simulink model "FlightController_1"  (R2022a)
settings: Solver=FixedStepAuto  StartTime=0.0  StopTime=inf  RelTol=1e-3
model workspace (MATLAB code in the model file):
  | m = 1.2;                  % mass (kg)
  | g = 9.81;                 % gravity (m/s^2)
  | I = diag([0.014,0.018,0.028]); % inertia matrix (kg·m^2)
  | l = 0.225;                % arm length (m)
  | b = 2.98e-6*(2*pi)^2;     % thrust coeff
  | d = 1.14e-7*(2*pi)^2;     % torque coeff
  | Cd = 0.1;                 % drag coeff
  | m_e = [20; 0; -40];       % earth mag field (uT)
  | wind = [0.5; 0; 0];       % constant wind (m/s)
libraries: slpidlib x6, simulink x3
settings Model: Creator=pvsha  LastModifiedBy=parv6
settings OptimizationCC: DefaultParameterBehavior=Inlined  EnhancedBackFolding=on  PassReuseOutputArgsThreshold=0  OptimizeBlockOrder=speed  DifferentSizesBufferReuse=on  OptimizationCustomize=off
settings DebuggingCC: UnderspecifiedInitializationDetection=Classic  ParameterTunabilityLossMsg=error  SFUnexpectedBacktrackingDiag=warning  SFNoUnconditionalDefaultTransitionDiag=warning
settings HardwareCC: TargetBitPerPointer=64  TargetBitPerSizeT=64  TargetBitPerPtrDiffT=64  TargetLongLongMode=on  TargetIntDivRoundTo=Zero  TargetEndianess=LittleEndian  TargetWordSize=64  TargetHWDeviceType=MATLAB Host  ProdEqTarget=off
settings ModelReferenceCC: PropagateSignalLabelsOutOfModel=off
settings SFSimCC: MATLABDynamicMemAlloc=off
settings RTWCC: Description=Generic Real-Time Target  GenCodeOnly=on  GenerateReport=on  BuildConfiguration=Debug  LaunchReport=on
settings CodeAppCC: ForceParamTrailComments=on  OperatorAnnotations=on  EnableCustomComments=on

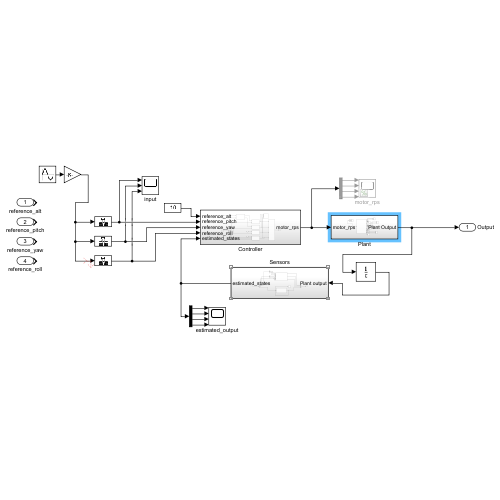
[thumbnail: Simulink's stored preview of the top-level diagram]
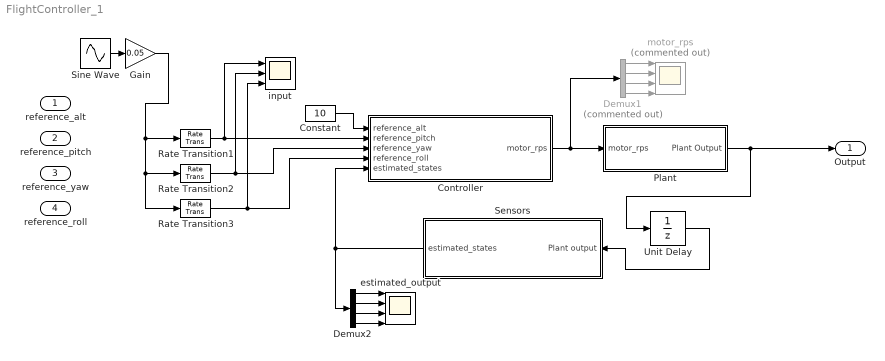
== system FlightController_1 ==
  reference_alt : Inport
  reference_pitch : Inport  Port=2
  reference_yaw : Inport  Port=3
  reference_roll : Inport  Port=4
  Constant : Constant  Value=10
  Controller : Subsystem
  Demux1 : Demux  Commented=on
  Demux2 : Demux
  Gain : Gain  Gain=0.05
  Plant : Subsystem
  Rate Transition1 : RateTransition  OutPortSampleTime=0.1
  Rate Transition2 : RateTransition  OutPortSampleTime=0.1
  Rate Transition3 : RateTransition  OutPortSampleTime=0.1
  Sensors : Subsystem
  Sine Wave : Sin  SampleTime=0
  Unit Delay : UnitDelay  SampleTime=-1  HasFrameUpgradeWarning=on
  estimated_output : Scope  NumInputPorts=4
  input : Scope  NumInputPorts=3
  motor_rps : Scope  Commented=on  NumInputPorts=4
  Output : Outport  SignalName=Output
  wires:
  Sensors/1(estimated_states) -> Demux2/1, Controller/5(estimated_states)
  Plant/1(Plant Output) -> Unit Delay/1, Output/1
  Rate Transition1/1 -> input/1, Controller/2(reference_pitch)
  Rate Transition2/1 -> input/2, Controller/3(reference_yaw)
  Rate Transition3/1 -> input/3, Controller/4(reference_roll)
  Unit Delay/1 -> Sensors/1(Plant output)
  Gain/1 -> Rate Transition3/1, Rate Transition2/1, Rate Transition1/1
  Demux1/1 -> motor_rps/1
  Demux1/3 -> motor_rps/3
  Demux1/4 -> motor_rps/4
  Demux1/2 -> motor_rps/2
  Controller/1(motor_rps) -> Demux1/1, Plant/1(motor_rps)
  Demux2/1 -> estimated_output/1
  Demux2/3 -> estimated_output/3
  Demux2/4 -> estimated_output/4
  Demux2/2 -> estimated_output/2
  Sine Wave/1 -> Gain/1
  ? -> ?
  Constant/1 -> Controller/1(reference_alt)

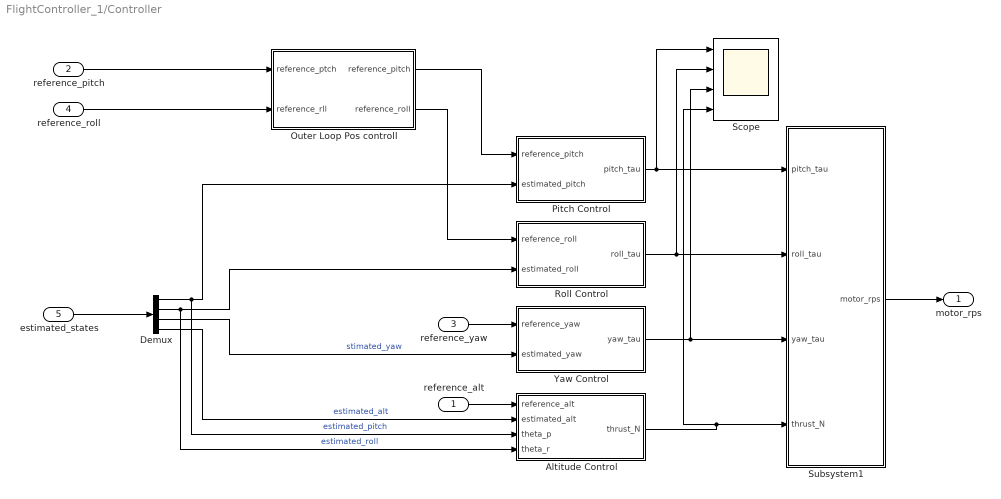
== system FlightController_1/Controller ==
  reference_alt : Inport
  reference_pitch : Inport  Port=2
  reference_yaw : Inport  Port=3
  reference_roll : Inport  Port=4
  estimated_states : Inport  Port=5  PortDimensions=4
  Altitude Control : Subsystem
  Demux : Demux
  Outer Loop Pos controll : Subsystem
  Pitch Control : Subsystem
  Roll Control : Subsystem
  Scope : Scope  NumInputPorts=4
  Subsystem1 : Subsystem
  Yaw Control : Subsystem
  motor_rps : Outport
  wires:
  estimated_states/1 -> Demux/1
  Subsystem1/1(motor_rps) -> motor_rps/1
  Pitch Control/1(pitch_tau) -> Scope/1, Subsystem1/1(pitch_tau)
  Roll Control/1(roll_tau) -> Scope/2, Subsystem1/2(roll_tau)
  Altitude Control/1(thrust_N) -> Scope/4, Subsystem1/4(thrust_N)
  reference_yaw/1 -> Yaw Control/1(reference_yaw)
  reference_pitch/1 -> Outer Loop Pos controll/1(reference_ptch)
  reference_alt/1 -> Altitude Control/1(reference_alt)
  Demux/4 -> Altitude Control/2(estimated_alt)  "estimated_alt"
  Demux/1 -> Altitude Control/3(theta_p), Pitch Control/2(estimated_pitch)  "estimated_pitch"
  Demux/2 -> Altitude Control/4(theta_r), Roll Control/2(estimated_roll)  "estimated_roll"
  Demux/3 -> Yaw Control/2(estimated_yaw)  "stimated_yaw"
  Outer Loop Pos controll/1(reference_pitch) -> Pitch Control/1(reference_pitch)
  Outer Loop Pos controll/2(reference_roll) -> Roll Control/1(reference_roll)
  reference_roll/1 -> Outer Loop Pos controll/2(reference_rll)
  Yaw Control/1(yaw_tau) -> Scope/3, Subsystem1/3(yaw_tau)

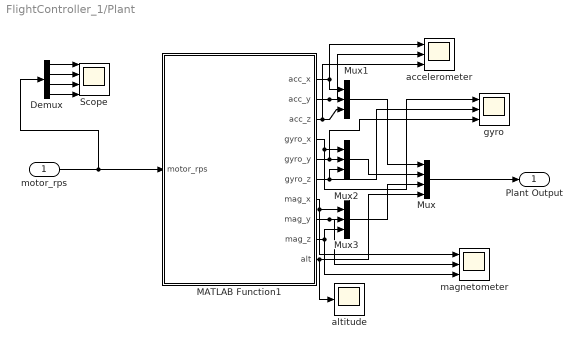
== system FlightController_1/Plant ==
  motor_rps : Inport
  Demux : Demux
  MATLAB Function1 : MATLAB Function  TreatAsAtomicUnit=on
  Mux : Mux
  Mux1 : Mux  Inputs=3
  Mux2 : Mux  Inputs=3
  Mux3 : Mux  Inputs=3
  Scope : Scope  NumInputPorts=4
  accelerometer : Scope  NumInputPorts=3
  altitude : Scope
  gyro : Scope  NumInputPorts=3
  magnetometer : Scope  NumInputPorts=3
  Plant Output : Outport
  wires:
  Mux/1 -> Plant Output/1
  motor_rps/1 -> MATLAB Function1/1(motor_rps), Demux/1
  Demux/1 -> Scope/1
  Demux/2 -> Scope/2
  Demux/3 -> Scope/3
  Demux/4 -> Scope/4
  MATLAB Function1/2(acc_y) -> accelerometer/2, Mux1/2
  MATLAB Function1/1(acc_x) -> accelerometer/1, Mux1/1
  MATLAB Function1/3(acc_z) -> Mux1/3, accelerometer/3
  MATLAB Function1/8(mag_y) -> magnetometer/2, Mux3/2
  MATLAB Function1/7(mag_x) -> magnetometer/1, Mux3/1
  MATLAB Function1/9(mag_z) -> magnetometer/3, Mux3/3
  Mux1/1 -> Mux/1
  Mux2/1 -> Mux/2
  Mux3/1 -> Mux/3
  MATLAB Function1/10(alt) -> Mux/4, altitude/1
  MATLAB Function1/6(gyro_z) -> gyro/2, Mux2/3
  MATLAB Function1/4(gyro_x) -> gyro/1, Mux2/1
  MATLAB Function1/5(gyro_y) -> gyro/3, Mux2/2

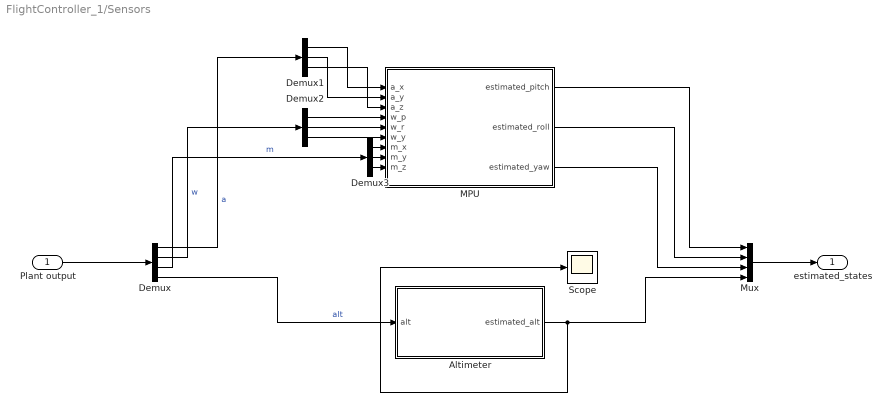
== system FlightController_1/Sensors ==
  Plant output : Inport
  Altimeter : Subsystem
  Demux : Demux
  Demux1 : Demux  Outputs=3
  Demux2 : Demux  Outputs=3
  Demux3 : Demux  Outputs=3
  MPU : Subsystem
  Mux : Mux
  Scope : Scope
  estimated_states : Outport
  wires:
  Plant output/1 -> Demux/1
  MPU/2(estimated_roll) -> Mux/2
  MPU/3(estimated_yaw) -> Mux/3
  MPU/1(estimated_pitch) -> Mux/1
  Mux/1 -> estimated_states/1
  Altimeter/1(estimated_alt) -> Scope/1, Mux/4
  Demux/1 -> Demux1/1  "a"
  Demux1/1 -> MPU/1(a_x)
  Demux1/2 -> MPU/2(a_y)
  Demux1/3 -> MPU/3(a_z)
  Demux2/2 -> MPU/5(w_r)
  Demux2/1 -> MPU/4(w_p)
  Demux2/3 -> MPU/6(w_y)
  Demux/2 -> Demux2/1  "w"
  Demux3/1 -> MPU/7(m_x)
  Demux3/2 -> MPU/8(m_y)
  Demux3/3 -> MPU/9(m_z)
  Demux/3 -> Demux3/1  "m"
  Demux/4 -> Altimeter/1(alt)  "alt"

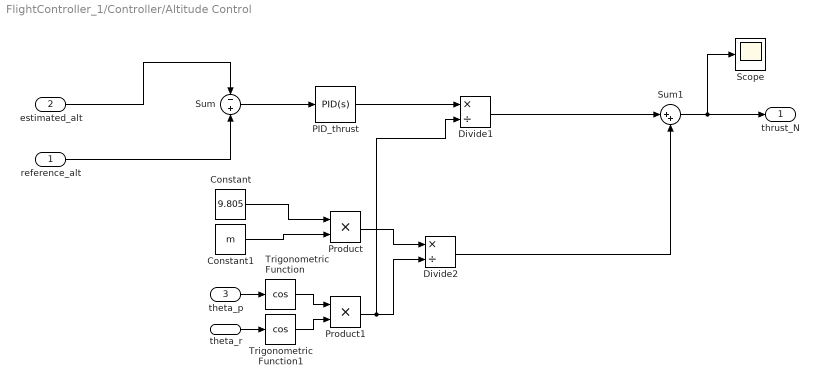
== system FlightController_1/Controller/Altitude Control ==
  reference_alt : Inport
  estimated_alt : Inport  Port=2
  theta_p : Inport  Port=3
  theta_r : Inport  Port=4
  Constant : Constant  Value=9.805
  Constant1 : Constant  Value=m
  Divide1 : Product  Inputs=*/
  Divide2 : Product  Inputs=*/
  PID_thrust : slpidlib/PID Controller  Controller=PID  Form=Parallel  TimeDomain=Continuous-time  UseExternalTs=off  SampleTime=-1  IntegratorMethod=Forward Euler  FilterMethod=Forward Euler  ControllerParametersSource=internal  P=0.8  I=0.5  UseKiTs=off  D=0  N=100  UseFilter=on  TunerSelectOption=Transfer Function Based (PID Tuner App)  InitialConditionSource=internal  InitialConditionForIntegrator=0  InitialConditionForFilter=0  DifferentiatorICPrevScaledInput=0  ExternalReset=none  TrackingMode=off  Kt=1  LimitOutput=off  SatLimitsSource=internal  UpperSaturationLimit=inf  LowerSaturationLimit=-inf  LinearizeAsGain=on  AntiWindupMode=none  Kb=1  POutMin=[]  POutMax=[]  IOutMin=[]  IOutMax=[]  DOutMin=[]  DOutMax=[]  NOutMin=[]  NOutMax=[]  SumOutMin=[]  SumOutMax=[]  SaturationOutMin=[]  SaturationOutMax=[]  PParamMin=[]  PParamMax=[]  IParamMin=[]  IParamMax=[]  DParamMin=[]  DParamMax=[]  NParamMin=[]  NParamMax=[]  KbParamMin=[]  KbParamMax=[]  KtParamMin=[]  KtParamMax=[]  KbOutMin=[]  KbOutMax=[]  KtOutMin=[]  KtOutMax=[]  IntegratorOutMin=[]  IntegratorOutMax=[]  FilterOutMin=[]  FilterOutMax=[]  SumI1OutMin=[]  SumI1OutMax=[]  SumI2OutMin=[]  SumI2OutMax=[]  SumI3OutMin=[]  SumI3OutMax=[]  SumI4OutMin=[]  SumI4OutMax=[]  SumDOutMin=[]  SumDOutMax=[]  DifferentiatorOutMin=[]  DifferentiatorOutMax=[]  FilterDiffOutCoefMin=[]  FilterDiffOutCoefMax=[]  ReciprocalOutMin=[]  ReciprocalOutMax=[]  SumDenOutMin=[]  SumDenOutMax=[]  SumNumOutMin=[]  SumNumOutMax=[]  DivideOutMin=[]  DivideOutMax=[]  UdiffTsProdOutMin=[]  UdiffTsProdOutMax=[]  NTsProdOutMin=[]  NTsProdOutMax=[]  UintegralTsProdOutMin=[]  UintegralTsProdOutMax=[]  UngainTsProdOutMin=[]  UngainTsProdOutMax=[]  ClampingZeroOutDataTypeStr=Inherit: Inherit via back propagation  ClampingZeroOutMin=[]  ClampingZeroOutMax=[]  FilterDenConstantOutDataTypeStr=Inherit: Inherit via back propagation  FilterDenConstantOutMin=[]  FilterDenConstantOutMax=[]  PCopyOutDataTypeStr=Inherit: Inherit via back propagation  PCopyOutMin=[]  PCopyOutMax=[]  NCopyOutDataTypeStr=Inherit: Inherit via back propagation  NCopyOutMin=[]  NCopyOutMax=[]  IntegratorContinuousStateAttributes=''  IntegratorStateMustResolveToSignalObject=off  IntegratorRTWStateStorageClass=Auto  FilterContinuousStateAttributes=''  FilterStateMustResolveToSignalObject=off  FilterRTWStateStorageClass=Auto  ParallelPVariant=InternalParameters  IdealPVariant=Disabled  IVariant=InternalParameters  DVariant=InternalParameters  IntegratorVariant=Continuous  SatVariant=Disabled  AWVariant=Passthrough  PCopyVariant=Disabled  TRVariant=Disabled  FdbkBlocksVariant=Forward  IdealPFdbkVariant=Disabled  SatFdbkVariant=Disabled  DerivativeFilterVariant=ContFilter  NVariant=InternalParameters  NCopyVariant=Disabled  FilterICVariant=InternalICsFilter  IntegratorICVariant=InternalICs  ExternalResetVariant=Disabled  TRSumVariant=Passthrough  SumFdbkVariant=Disabled  SumVariant=Sum_PID  TsampFilterVariant=InternalTs  TsampNgainVariant=Passthrough  TsampIntegralVariant=Passthrough  ExternalSaturationOutDataTypeStr=Inherit: Same as second input  aMode=0
  Product : Product
  Product1 : Product
  Scope : Scope
  Sum : Sum  Inputs=-+
  Sum1 : Sum  Inputs=|++
  Trigonometric Function : Trigonometry  Operator=cos
  Trigonometric Function1 : Trigonometry  Operator=cos
  thrust_N : Outport
  wires:
  estimated_alt/1 -> Sum/1
  Sum/1 -> PID_thrust/1
  reference_alt/1 -> Sum/2
  Constant1/1 -> Product/2
  Constant/1 -> Product/1
  Product/1 -> Divide2/1
  Product1/1 -> Divide2/2, Divide1/2
  Divide2/1 -> Sum1/2
  PID_thrust/1 -> Divide1/1
  Divide1/1 -> Sum1/1
  theta_r/1 -> Trigonometric Function1/1
  Trigonometric Function1/1 -> Product1/2
  theta_p/1 -> Trigonometric Function/1
  Trigonometric Function/1 -> Product1/1
  Sum1/1 -> Scope/1, thrust_N/1

== system FlightController_1/Controller/Outer Loop Pos controll ==
  reference_ptch : Inport
  reference_rll : Inport  Port=2
  PID_pitch : slpidlib/PID Controller  Commented=on  Controller=PID  Form=Parallel  TimeDomain=Continuous-time  UseExternalTs=off  SampleTime=-1  IntegratorMethod=Forward Euler  FilterMethod=Forward Euler  ControllerParametersSource=internal  P=1  I=1  UseKiTs=off  D=0  N=100  UseFilter=on  TunerSelectOption=Transfer Function Based (PID Tuner App)  InitialConditionSource=internal  InitialConditionForIntegrator=0  InitialConditionForFilter=0  DifferentiatorICPrevScaledInput=0  ExternalReset=none  TrackingMode=off  Kt=1  LimitOutput=off  SatLimitsSource=internal  UpperSaturationLimit=inf  LowerSaturationLimit=-inf  LinearizeAsGain=on  AntiWindupMode=none  Kb=1  POutMin=[]  POutMax=[]  IOutMin=[]  IOutMax=[]  DOutMin=[]  DOutMax=[]  NOutMin=[]  NOutMax=[]  SumOutMin=[]  SumOutMax=[]  SaturationOutMin=[]  SaturationOutMax=[]  PParamMin=[]  PParamMax=[]  IParamMin=[]  IParamMax=[]  DParamMin=[]  DParamMax=[]  NParamMin=[]  NParamMax=[]  KbParamMin=[]  KbParamMax=[]  KtParamMin=[]  KtParamMax=[]  KbOutMin=[]  KbOutMax=[]  KtOutMin=[]  KtOutMax=[]  IntegratorOutMin=[]  IntegratorOutMax=[]  FilterOutMin=[]  FilterOutMax=[]  SumI1OutMin=[]  SumI1OutMax=[]  SumI2OutMin=[]  SumI2OutMax=[]  SumI3OutMin=[]  SumI3OutMax=[]  SumI4OutMin=[]  SumI4OutMax=[]  SumDOutMin=[]  SumDOutMax=[]  DifferentiatorOutMin=[]  DifferentiatorOutMax=[]  FilterDiffOutCoefMin=[]  FilterDiffOutCoefMax=[]  ReciprocalOutMin=[]  ReciprocalOutMax=[]  SumDenOutMin=[]  SumDenOutMax=[]  SumNumOutMin=[]  SumNumOutMax=[]  DivideOutMin=[]  DivideOutMax=[]  UdiffTsProdOutMin=[]  UdiffTsProdOutMax=[]  NTsProdOutMin=[]  NTsProdOutMax=[]  UintegralTsProdOutMin=[]  UintegralTsProdOutMax=[]  UngainTsProdOutMin=[]  UngainTsProdOutMax=[]  ClampingZeroOutDataTypeStr=Inherit: Inherit via back propagation  ClampingZeroOutMin=[]  ClampingZeroOutMax=[]  FilterDenConstantOutDataTypeStr=Inherit: Inherit via back propagation  FilterDenConstantOutMin=[]  FilterDenConstantOutMax=[]  PCopyOutDataTypeStr=Inherit: Inherit via back propagation  PCopyOutMin=[]  PCopyOutMax=[]  NCopyOutDataTypeStr=Inherit: Inherit via back propagation  NCopyOutMin=[]  NCopyOutMax=[]  IntegratorContinuousStateAttributes=''  IntegratorStateMustResolveToSignalObject=off  IntegratorRTWStateStorageClass=Auto  FilterContinuousStateAttributes=''  FilterStateMustResolveToSignalObject=off  FilterRTWStateStorageClass=Auto  ParallelPVariant=InternalParameters  IdealPVariant=Disabled  IVariant=InternalParameters  DVariant=InternalParameters  IntegratorVariant=Continuous  SatVariant=Disabled  AWVariant=Passthrough  PCopyVariant=Disabled  TRVariant=Disabled  FdbkBlocksVariant=Forward  IdealPFdbkVariant=Disabled  SatFdbkVariant=Disabled  DerivativeFilterVariant=ContFilter  NVariant=InternalParameters  NCopyVariant=Disabled  FilterICVariant=InternalICsFilter  IntegratorICVariant=InternalICs  ExternalResetVariant=Disabled  TRSumVariant=Passthrough  SumFdbkVariant=Disabled  SumVariant=Sum_PID  TsampFilterVariant=InternalTs  TsampNgainVariant=Passthrough  TsampIntegralVariant=Passthrough  ExternalSaturationOutDataTypeStr=Inherit: Same as second input  aMode=0
  PID_roll : slpidlib/PID Controller  Commented=on  Controller=PID  Form=Parallel  TimeDomain=Continuous-time  UseExternalTs=off  SampleTime=-1  IntegratorMethod=Forward Euler  FilterMethod=Forward Euler  ControllerParametersSource=internal  P=1  I=1  UseKiTs=off  D=0  N=100  UseFilter=on  TunerSelectOption=Transfer Function Based (PID Tuner App)  InitialConditionSource=internal  InitialConditionForIntegrator=0  InitialConditionForFilter=0  DifferentiatorICPrevScaledInput=0  ExternalReset=none  TrackingMode=off  Kt=1  LimitOutput=off  SatLimitsSource=internal  UpperSaturationLimit=inf  LowerSaturationLimit=-inf  LinearizeAsGain=on  AntiWindupMode=none  Kb=1  POutMin=[]  POutMax=[]  IOutMin=[]  IOutMax=[]  DOutMin=[]  DOutMax=[]  NOutMin=[]  NOutMax=[]  SumOutMin=[]  SumOutMax=[]  SaturationOutMin=[]  SaturationOutMax=[]  PParamMin=[]  PParamMax=[]  IParamMin=[]  IParamMax=[]  DParamMin=[]  DParamMax=[]  NParamMin=[]  NParamMax=[]  KbParamMin=[]  KbParamMax=[]  KtParamMin=[]  KtParamMax=[]  KbOutMin=[]  KbOutMax=[]  KtOutMin=[]  KtOutMax=[]  IntegratorOutMin=[]  IntegratorOutMax=[]  FilterOutMin=[]  FilterOutMax=[]  SumI1OutMin=[]  SumI1OutMax=[]  SumI2OutMin=[]  SumI2OutMax=[]  SumI3OutMin=[]  SumI3OutMax=[]  SumI4OutMin=[]  SumI4OutMax=[]  SumDOutMin=[]  SumDOutMax=[]  DifferentiatorOutMin=[]  DifferentiatorOutMax=[]  FilterDiffOutCoefMin=[]  FilterDiffOutCoefMax=[]  ReciprocalOutMin=[]  ReciprocalOutMax=[]  SumDenOutMin=[]  SumDenOutMax=[]  SumNumOutMin=[]  SumNumOutMax=[]  DivideOutMin=[]  DivideOutMax=[]  UdiffTsProdOutMin=[]  UdiffTsProdOutMax=[]  NTsProdOutMin=[]  NTsProdOutMax=[]  UintegralTsProdOutMin=[]  UintegralTsProdOutMax=[]  UngainTsProdOutMin=[]  UngainTsProdOutMax=[]  ClampingZeroOutDataTypeStr=Inherit: Inherit via back propagation  ClampingZeroOutMin=[]  ClampingZeroOutMax=[]  FilterDenConstantOutDataTypeStr=Inherit: Inherit via back propagation  FilterDenConstantOutMin=[]  FilterDenConstantOutMax=[]  PCopyOutDataTypeStr=Inherit: Inherit via back propagation  PCopyOutMin=[]  PCopyOutMax=[]  NCopyOutDataTypeStr=Inherit: Inherit via back propagation  NCopyOutMin=[]  NCopyOutMax=[]  IntegratorContinuousStateAttributes=''  IntegratorStateMustResolveToSignalObject=off  IntegratorRTWStateStorageClass=Auto  FilterContinuousStateAttributes=''  FilterStateMustResolveToSignalObject=off  FilterRTWStateStorageClass=Auto  ParallelPVariant=InternalParameters  IdealPVariant=Disabled  IVariant=InternalParameters  DVariant=InternalParameters  IntegratorVariant=Continuous  SatVariant=Disabled  AWVariant=Passthrough  PCopyVariant=Disabled  TRVariant=Disabled  FdbkBlocksVariant=Forward  IdealPFdbkVariant=Disabled  SatFdbkVariant=Disabled  DerivativeFilterVariant=ContFilter  NVariant=InternalParameters  NCopyVariant=Disabled  FilterICVariant=InternalICsFilter  IntegratorICVariant=InternalICs  ExternalResetVariant=Disabled  TRSumVariant=Passthrough  SumFdbkVariant=Disabled  SumVariant=Sum_PID  TsampFilterVariant=InternalTs  TsampNgainVariant=Passthrough  TsampIntegralVariant=Passthrough  ExternalSaturationOutDataTypeStr=Inherit: Same as second input  aMode=0
  World to body conversion : Subsystem  Commented=on
  reference_pitch : Outport
  reference_roll : Outport  Port=2
  wires:
  World to body conversion/1(ref_pitch_b) -> ?
  World to body conversion/2(ref_roll_b) -> ?
  reference_ptch/1 -> reference_pitch/1
  reference_rll/1 -> reference_roll/1

== system FlightController_1/Controller/Pitch Control ==
  reference_pitch : Inport
  estimated_pitch : Inport  Port=2
  PID_pitch : slpidlib/PID Controller  Controller=PID  Form=Parallel  TimeDomain=Continuous-time  UseExternalTs=off  SampleTime=-1  IntegratorMethod=Forward Euler  FilterMethod=Forward Euler  ControllerParametersSource=internal  P=1  I=2  UseKiTs=off  D=0  N=100  UseFilter=on  TunerSelectOption=Transfer Function Based (PID Tuner App)  InitialConditionSource=internal  InitialConditionForIntegrator=0  InitialConditionForFilter=0  DifferentiatorICPrevScaledInput=0  ExternalReset=none  TrackingMode=off  Kt=1  LimitOutput=off  SatLimitsSource=internal  UpperSaturationLimit=inf  LowerSaturationLimit=-inf  LinearizeAsGain=on  AntiWindupMode=none  Kb=1  POutMin=[]  POutMax=[]  IOutMin=[]  IOutMax=[]  DOutMin=[]  DOutMax=[]  NOutMin=[]  NOutMax=[]  SumOutMin=[]  SumOutMax=[]  SaturationOutMin=[]  SaturationOutMax=[]  PParamMin=[]  PParamMax=[]  IParamMin=[]  IParamMax=[]  DParamMin=[]  DParamMax=[]  NParamMin=[]  NParamMax=[]  KbParamMin=[]  KbParamMax=[]  KtParamMin=[]  KtParamMax=[]  KbOutMin=[]  KbOutMax=[]  KtOutMin=[]  KtOutMax=[]  IntegratorOutMin=[]  IntegratorOutMax=[]  FilterOutMin=[]  FilterOutMax=[]  SumI1OutMin=[]  SumI1OutMax=[]  SumI2OutMin=[]  SumI2OutMax=[]  SumI3OutMin=[]  SumI3OutMax=[]  SumI4OutMin=[]  SumI4OutMax=[]  SumDOutMin=[]  SumDOutMax=[]  DifferentiatorOutMin=[]  DifferentiatorOutMax=[]  FilterDiffOutCoefMin=[]  FilterDiffOutCoefMax=[]  ReciprocalOutMin=[]  ReciprocalOutMax=[]  SumDenOutMin=[]  SumDenOutMax=[]  SumNumOutMin=[]  SumNumOutMax=[]  DivideOutMin=[]  DivideOutMax=[]  UdiffTsProdOutMin=[]  UdiffTsProdOutMax=[]  NTsProdOutMin=[]  NTsProdOutMax=[]  UintegralTsProdOutMin=[]  UintegralTsProdOutMax=[]  UngainTsProdOutMin=[]  UngainTsProdOutMax=[]  ClampingZeroOutDataTypeStr=Inherit: Inherit via back propagation  ClampingZeroOutMin=[]  ClampingZeroOutMax=[]  FilterDenConstantOutDataTypeStr=Inherit: Inherit via back propagation  FilterDenConstantOutMin=[]  FilterDenConstantOutMax=[]  PCopyOutDataTypeStr=Inherit: Inherit via back propagation  PCopyOutMin=[]  PCopyOutMax=[]  NCopyOutDataTypeStr=Inherit: Inherit via back propagation  NCopyOutMin=[]  NCopyOutMax=[]  IntegratorContinuousStateAttributes=''  IntegratorStateMustResolveToSignalObject=off  IntegratorRTWStateStorageClass=Auto  FilterContinuousStateAttributes=''  FilterStateMustResolveToSignalObject=off  FilterRTWStateStorageClass=Auto  ParallelPVariant=InternalParameters  IdealPVariant=Disabled  IVariant=InternalParameters  DVariant=InternalParameters  IntegratorVariant=Continuous  SatVariant=Disabled  AWVariant=Passthrough  PCopyVariant=Disabled  TRVariant=Disabled  FdbkBlocksVariant=Forward  IdealPFdbkVariant=Disabled  SatFdbkVariant=Disabled  DerivativeFilterVariant=ContFilter  NVariant=InternalParameters  NCopyVariant=Disabled  FilterICVariant=InternalICsFilter  IntegratorICVariant=InternalICs  ExternalResetVariant=Disabled  TRSumVariant=Passthrough  SumFdbkVariant=Disabled  SumVariant=Sum_PID  TsampFilterVariant=InternalTs  TsampNgainVariant=Passthrough  TsampIntegralVariant=Passthrough  ExternalSaturationOutDataTypeStr=Inherit: Same as second input  aMode=0
  Sum : Sum  Inputs=|+-
  pitch_tau : Outport
  wires:
  estimated_pitch/1 -> Sum/1
  reference_pitch/1 -> Sum/2
  Sum/1 -> PID_pitch/1
  PID_pitch/1 -> pitch_tau/1

== system FlightController_1/Controller/Roll Control ==
  reference_roll : Inport
  estimated_roll : Inport  Port=2
  PID_roll : slpidlib/PID Controller  Controller=PID  Form=Parallel  TimeDomain=Continuous-time  UseExternalTs=off  SampleTime=-1  IntegratorMethod=Forward Euler  FilterMethod=Forward Euler  ControllerParametersSource=internal  P=1  I=1  UseKiTs=off  D=0  N=100  UseFilter=on  TunerSelectOption=Transfer Function Based (PID Tuner App)  InitialConditionSource=internal  InitialConditionForIntegrator=0  InitialConditionForFilter=0  DifferentiatorICPrevScaledInput=0  ExternalReset=none  TrackingMode=off  Kt=1  LimitOutput=off  SatLimitsSource=internal  UpperSaturationLimit=inf  LowerSaturationLimit=-inf  LinearizeAsGain=on  AntiWindupMode=none  Kb=1  POutMin=[]  POutMax=[]  IOutMin=[]  IOutMax=[]  DOutMin=[]  DOutMax=[]  NOutMin=[]  NOutMax=[]  SumOutMin=[]  SumOutMax=[]  SaturationOutMin=[]  SaturationOutMax=[]  PParamMin=[]  PParamMax=[]  IParamMin=[]  IParamMax=[]  DParamMin=[]  DParamMax=[]  NParamMin=[]  NParamMax=[]  KbParamMin=[]  KbParamMax=[]  KtParamMin=[]  KtParamMax=[]  KbOutMin=[]  KbOutMax=[]  KtOutMin=[]  KtOutMax=[]  IntegratorOutMin=[]  IntegratorOutMax=[]  FilterOutMin=[]  FilterOutMax=[]  SumI1OutMin=[]  SumI1OutMax=[]  SumI2OutMin=[]  SumI2OutMax=[]  SumI3OutMin=[]  SumI3OutMax=[]  SumI4OutMin=[]  SumI4OutMax=[]  SumDOutMin=[]  SumDOutMax=[]  DifferentiatorOutMin=[]  DifferentiatorOutMax=[]  FilterDiffOutCoefMin=[]  FilterDiffOutCoefMax=[]  ReciprocalOutMin=[]  ReciprocalOutMax=[]  SumDenOutMin=[]  SumDenOutMax=[]  SumNumOutMin=[]  SumNumOutMax=[]  DivideOutMin=[]  DivideOutMax=[]  UdiffTsProdOutMin=[]  UdiffTsProdOutMax=[]  NTsProdOutMin=[]  NTsProdOutMax=[]  UintegralTsProdOutMin=[]  UintegralTsProdOutMax=[]  UngainTsProdOutMin=[]  UngainTsProdOutMax=[]  ClampingZeroOutDataTypeStr=Inherit: Inherit via back propagation  ClampingZeroOutMin=[]  ClampingZeroOutMax=[]  FilterDenConstantOutDataTypeStr=Inherit: Inherit via back propagation  FilterDenConstantOutMin=[]  FilterDenConstantOutMax=[]  PCopyOutDataTypeStr=Inherit: Inherit via back propagation  PCopyOutMin=[]  PCopyOutMax=[]  NCopyOutDataTypeStr=Inherit: Inherit via back propagation  NCopyOutMin=[]  NCopyOutMax=[]  IntegratorContinuousStateAttributes=''  IntegratorStateMustResolveToSignalObject=off  IntegratorRTWStateStorageClass=Auto  FilterContinuousStateAttributes=''  FilterStateMustResolveToSignalObject=off  FilterRTWStateStorageClass=Auto  ParallelPVariant=InternalParameters  IdealPVariant=Disabled  IVariant=InternalParameters  DVariant=InternalParameters  IntegratorVariant=Continuous  SatVariant=Disabled  AWVariant=Passthrough  PCopyVariant=Disabled  TRVariant=Disabled  FdbkBlocksVariant=Forward  IdealPFdbkVariant=Disabled  SatFdbkVariant=Disabled  DerivativeFilterVariant=ContFilter  NVariant=InternalParameters  NCopyVariant=Disabled  FilterICVariant=InternalICsFilter  IntegratorICVariant=InternalICs  ExternalResetVariant=Disabled  TRSumVariant=Passthrough  SumFdbkVariant=Disabled  SumVariant=Sum_PID  TsampFilterVariant=InternalTs  TsampNgainVariant=Passthrough  TsampIntegralVariant=Passthrough  ExternalSaturationOutDataTypeStr=Inherit: Same as second input  aMode=0
  Sum : Sum  Inputs=|+-
  roll_tau : Outport
  wires:
  estimated_roll/1 -> Sum/1
  reference_roll/1 -> Sum/2
  Sum/1 -> PID_roll/1
  PID_roll/1 -> roll_tau/1

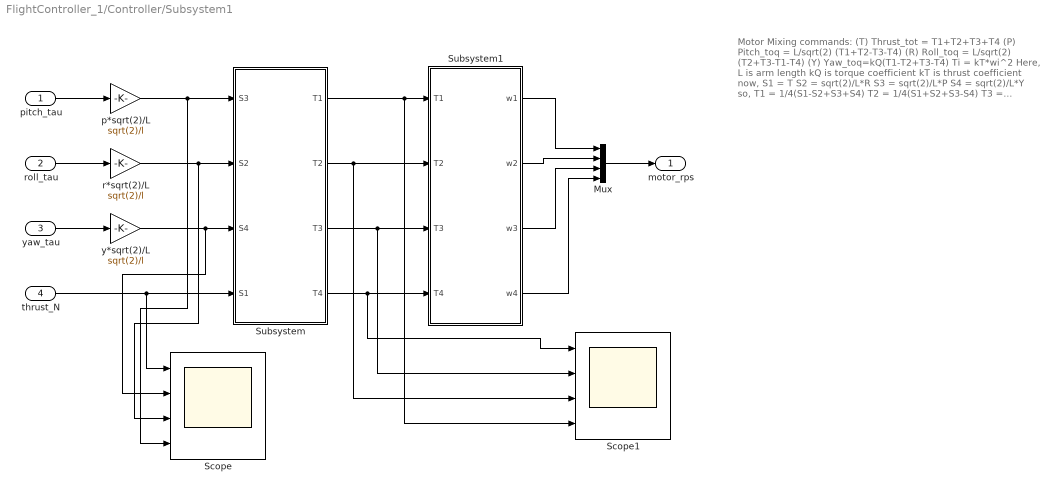
== system FlightController_1/Controller/Subsystem1 ==
  note: Motor Mixing commands:
      |
      | (T) Thrust_tot = T1+T2+T3+T4
      | (P) Pitch_toq = L/sqrt(2) (T1+T2-T3-T4)
      | (R) Roll_toq = L/sqrt(2) (T2+T3-T1-T4)
      | (Y) Yaw_toq=kQ(T1-T2+T3-T4)
      | Ti = kT*wi^2
      |
      | Here,
      | L is arm length
      | kQ is torque coefficient
      | kT is thrust coefficient
      |
      | now,
      | S1 = T
      | S2 = sqrt(2)/L*R
      | S3 = sqrt(2)/L*P
      | S4 = sqrt(2)/L*Y
      |
      | so,
      | T1 = 1/4(S1-S2+S3+S4)
      | T2 = 1/4(S1+S2+S3-S4)
      | T3 = 1/4(S1+S2-S3+S4)
      | T4 = 1/4(S1-S2-S3-S4)
      |
      | and ofcourse,
      | wi = sqrt(Ti/kT)
  pitch_tau : Inport
  roll_tau : Inport  Port=2
  yaw_tau : Inport  Port=3
  thrust_N : Inport  Port=4
  Mux : Mux
  Scope : Scope  NumInputPorts=4
  Scope1 : Scope  NumInputPorts=4
  Subsystem : Subsystem
  Subsystem1 : Subsystem
  p*sqrt(2)/L : Gain  Gain=sqrt(2)/l
  r*sqrt(2)/L : Gain  Gain=sqrt(2)/l
  y*sqrt(2)/L : Gain  Gain=sqrt(2)/l
  motor_rps : Outport
  wires:
  pitch_tau/1 -> p*sqrt(2)/L/1
  roll_tau/1 -> r*sqrt(2)/L/1
  yaw_tau/1 -> y*sqrt(2)/L/1
  p*sqrt(2)/L/1 -> Scope/4, Subsystem/1(S3)
  r*sqrt(2)/L/1 -> Scope/3, Subsystem/2(S2)
  y*sqrt(2)/L/1 -> Scope/2, Subsystem/3(S4)
  thrust_N/1 -> Subsystem/4(S1), Scope/1
  Subsystem/1(T1) -> Scope1/4, Subsystem1/1(T1)
  Subsystem/2(T2) -> Scope1/3, Subsystem1/2(T2)
  Subsystem/3(T3) -> Scope1/2, Subsystem1/3(T3)
  Subsystem/4(T4) -> Scope1/1, Subsystem1/4(T4)
  Subsystem1/1(w1) -> Mux/1
  Subsystem1/2(w2) -> Mux/2
  Subsystem1/3(w3) -> Mux/3
  Subsystem1/4(w4) -> Mux/4
  Mux/1 -> motor_rps/1

== system FlightController_1/Controller/Yaw Control ==
  reference_yaw : Inport
  estimated_yaw : Inport  Port=2
  PID_yaw : slpidlib/PID Controller  Controller=PID  Form=Parallel  TimeDomain=Continuous-time  UseExternalTs=off  SampleTime=-1  IntegratorMethod=Forward Euler  FilterMethod=Forward Euler  ControllerParametersSource=internal  P=1  I=1  UseKiTs=off  D=0  N=100  UseFilter=on  TunerSelectOption=Transfer Function Based (PID Tuner App)  InitialConditionSource=internal  InitialConditionForIntegrator=0  InitialConditionForFilter=0  DifferentiatorICPrevScaledInput=0  ExternalReset=none  TrackingMode=off  Kt=1  LimitOutput=off  SatLimitsSource=internal  UpperSaturationLimit=inf  LowerSaturationLimit=-inf  LinearizeAsGain=on  AntiWindupMode=none  Kb=1  POutMin=[]  POutMax=[]  IOutMin=[]  IOutMax=[]  DOutMin=[]  DOutMax=[]  NOutMin=[]  NOutMax=[]  SumOutMin=[]  SumOutMax=[]  SaturationOutMin=[]  SaturationOutMax=[]  PParamMin=[]  PParamMax=[]  IParamMin=[]  IParamMax=[]  DParamMin=[]  DParamMax=[]  NParamMin=[]  NParamMax=[]  KbParamMin=[]  KbParamMax=[]  KtParamMin=[]  KtParamMax=[]  KbOutMin=[]  KbOutMax=[]  KtOutMin=[]  KtOutMax=[]  IntegratorOutMin=[]  IntegratorOutMax=[]  FilterOutMin=[]  FilterOutMax=[]  SumI1OutMin=[]  SumI1OutMax=[]  SumI2OutMin=[]  SumI2OutMax=[]  SumI3OutMin=[]  SumI3OutMax=[]  SumI4OutMin=[]  SumI4OutMax=[]  SumDOutMin=[]  SumDOutMax=[]  DifferentiatorOutMin=[]  DifferentiatorOutMax=[]  FilterDiffOutCoefMin=[]  FilterDiffOutCoefMax=[]  ReciprocalOutMin=[]  ReciprocalOutMax=[]  SumDenOutMin=[]  SumDenOutMax=[]  SumNumOutMin=[]  SumNumOutMax=[]  DivideOutMin=[]  DivideOutMax=[]  UdiffTsProdOutMin=[]  UdiffTsProdOutMax=[]  NTsProdOutMin=[]  NTsProdOutMax=[]  UintegralTsProdOutMin=[]  UintegralTsProdOutMax=[]  UngainTsProdOutMin=[]  UngainTsProdOutMax=[]  ClampingZeroOutDataTypeStr=Inherit: Inherit via back propagation  ClampingZeroOutMin=[]  ClampingZeroOutMax=[]  FilterDenConstantOutDataTypeStr=Inherit: Inherit via back propagation  FilterDenConstantOutMin=[]  FilterDenConstantOutMax=[]  PCopyOutDataTypeStr=Inherit: Inherit via back propagation  PCopyOutMin=[]  PCopyOutMax=[]  NCopyOutDataTypeStr=Inherit: Inherit via back propagation  NCopyOutMin=[]  NCopyOutMax=[]  IntegratorContinuousStateAttributes=''  IntegratorStateMustResolveToSignalObject=off  IntegratorRTWStateStorageClass=Auto  FilterContinuousStateAttributes=''  FilterStateMustResolveToSignalObject=off  FilterRTWStateStorageClass=Auto  ParallelPVariant=InternalParameters  IdealPVariant=Disabled  IVariant=InternalParameters  DVariant=InternalParameters  IntegratorVariant=Continuous  SatVariant=Disabled  AWVariant=Passthrough  PCopyVariant=Disabled  TRVariant=Disabled  FdbkBlocksVariant=Forward  IdealPFdbkVariant=Disabled  SatFdbkVariant=Disabled  DerivativeFilterVariant=ContFilter  NVariant=InternalParameters  NCopyVariant=Disabled  FilterICVariant=InternalICsFilter  IntegratorICVariant=InternalICs  ExternalResetVariant=Disabled  TRSumVariant=Passthrough  SumFdbkVariant=Disabled  SumVariant=Sum_PID  TsampFilterVariant=InternalTs  TsampNgainVariant=Passthrough  TsampIntegralVariant=Passthrough  ExternalSaturationOutDataTypeStr=Inherit: Same as second input  aMode=0
  Sum : Sum  Inputs=|+-
  yaw_tau : Outport
  wires:
  estimated_yaw/1 -> Sum/1
  PID_yaw/1 -> yaw_tau/1
  reference_yaw/1 -> Sum/2
  Sum/1 -> PID_yaw/1

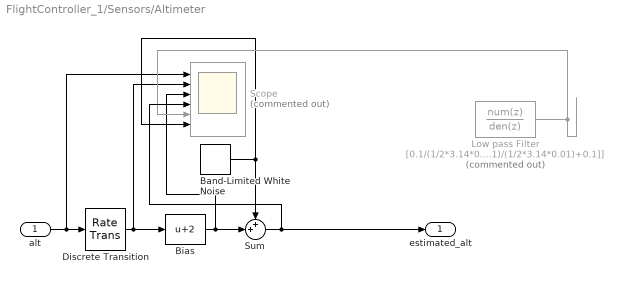
== system FlightController_1/Sensors/Altimeter ==
  alt : Inport
  Band-Limited White Noise : simulink/Sources/Band-Limited White Noise  Cov=[1]  Ts=0.1  seed=[23341]
  Bias : Bias  Bias=2  SaturateOnIntegerOverflow=off
  Discrete Transition : RateTransition  InitialCondition=0.1
  Low pass Filter : DiscreteFilter  Commented=on  Numerator=[0.1/(1/2*3.14*0.01)+0.1]  Denominator=[1 -[(1/2*3.14*0.01)/(1/2*3.14*0.01)+0.1]]
  Scope : Scope  Commented=on  NumInputPorts=6
  Sum : Sum  Inputs=++|
  estimated_alt : Outport
  wires:
  alt/1 -> Scope/1, Discrete Transition/1
  Discrete Transition/1 -> Scope/2, Bias/1
  Bias/1 -> Scope/3, Sum/2
  Band-Limited White Noise/1 -> Scope/6, Sum/1
  Low pass Filter/1 -> Scope/5
  Sum/1 -> estimated_alt/1, Scope/4

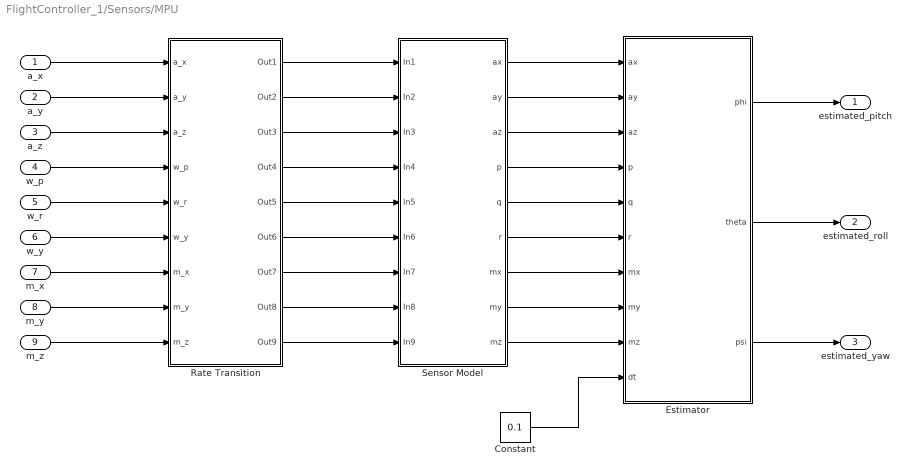
== system FlightController_1/Sensors/MPU ==
  a_x : Inport
  a_y : Inport  Port=2
  a_z : Inport  Port=3
  w_p : Inport  Port=4
  w_r : Inport  Port=5
  w_y : Inport  Port=6
  m_x : Inport  Port=7
  m_y : Inport  Port=8
  m_z : Inport  Port=9
  Constant : Constant  Value=0.1
  Estimator : MATLAB Function  TreatAsAtomicUnit=on
  Rate Transition : Subsystem
  Sensor Model : Subsystem
  estimated_pitch : Outport
  estimated_roll : Outport  Port=2
  estimated_yaw : Outport  Port=3
  wires:
  Sensor Model/1(ax) -> Estimator/1(ax)
  Sensor Model/2(ay) -> Estimator/2(ay)
  Sensor Model/3(az) -> Estimator/3(az)
  Sensor Model/4(p) -> Estimator/4(p)
  Sensor Model/5(q) -> Estimator/5(q)
  Sensor Model/6(r) -> Estimator/6(r)
  Sensor Model/7(mx) -> Estimator/7(mx)
  Sensor Model/8(my) -> Estimator/8(my)
  Sensor Model/9(mz) -> Estimator/9(mz)
  Rate Transition/1(Out1) -> Sensor Model/1(In1)
  Rate Transition/2(Out2) -> Sensor Model/2(In2)
  Rate Transition/3(Out3) -> Sensor Model/3(In3)
  Rate Transition/4(Out4) -> Sensor Model/4(In4)
  Rate Transition/5(Out5) -> Sensor Model/5(In5)
  Rate Transition/6(Out6) -> Sensor Model/6(In6)
  Rate Transition/7(Out7) -> Sensor Model/7(In7)
  Rate Transition/8(Out8) -> Sensor Model/8(In8)
  Rate Transition/9(Out9) -> Sensor Model/9(In9)
  a_x/1 -> Rate Transition/1(a_x)
  a_y/1 -> Rate Transition/2(a_y)
  a_z/1 -> Rate Transition/3(a_z)
  w_p/1 -> Rate Transition/4(w_p)
  w_r/1 -> Rate Transition/5(w_r)
  w_y/1 -> Rate Transition/6(w_y)
  m_x/1 -> Rate Transition/7(m_x)
  m_y/1 -> Rate Transition/8(m_y)
  m_z/1 -> Rate Transition/9(m_z)
  Estimator/1(phi) -> estimated_pitch/1
  Estimator/2(theta) -> estimated_roll/1
  Estimator/3(psi) -> estimated_yaw/1
  Constant/1 -> Estimator/10(dt)

== system FlightController_1/Controller/Outer Loop Pos controll/World to body conversion ==
  ref_pitch_w : Inport
  est_yaw_w : Inport  Port=2
  ref_roll_w : Inport  Port=3
  ref_pitch_b : Outport
  ref_roll_b : Outport  Port=2

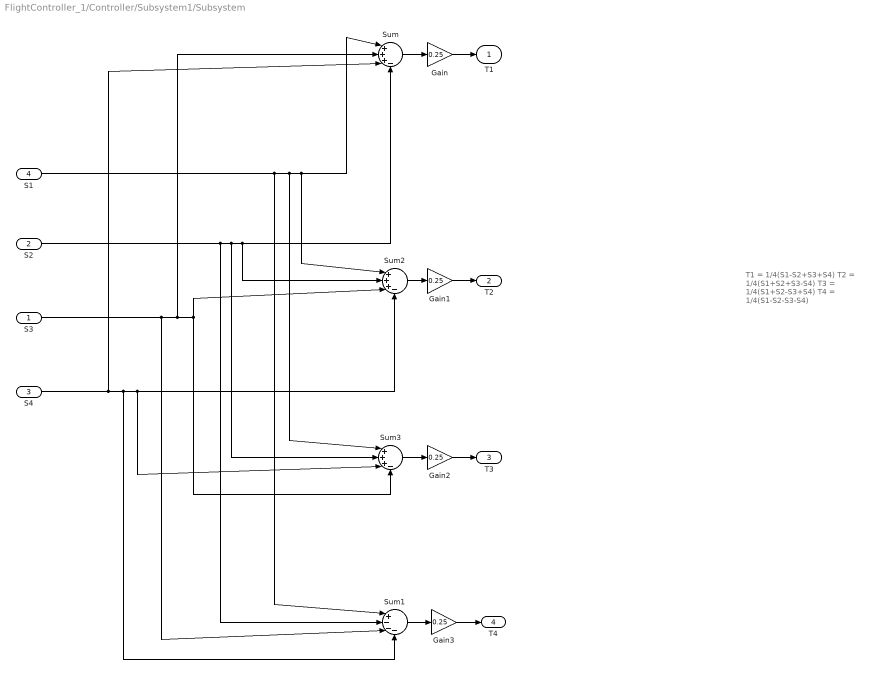
== system FlightController_1/Controller/Subsystem1/Subsystem ==
  note: T1 = 1/4(S1-S2+S3+S4)
      | T2 = 1/4(S1+S2+S3-S4)
      | T3 = 1/4(S1+S2-S3+S4)
      | T4 = 1/4(S1-S2-S3-S4)
  S3 : Inport
  S2 : Inport  Port=2
  S4 : Inport  Port=3
  S1 : Inport  Port=4
  Gain{,1..3} (4 alike) : Gain  Gain=0.25
  Sum : Sum  Inputs=|+++-
  Sum1 : Sum  Inputs=|+---
  Sum2 : Sum  Inputs=|+++-
  Sum3 : Sum  Inputs=|+++-
  T1 : Outport
  T2 : Outport  Port=2
  T3 : Outport  Port=3
  T4 : Outport  Port=4
  wires:
  Gain3/1 -> T4/1
  Gain2/1 -> T3/1
  Gain1/1 -> T2/1
  Gain/1 -> T1/1
  S1/1 -> Sum/1, Sum2/1, Sum3/1, Sum1/1
  S3/1 -> Sum1/3, Sum3/4, Sum2/3, Sum/2
  S4/1 -> Sum/3, Sum1/4, Sum3/3, Sum2/4
  S2/1 -> Sum1/2, Sum/4, Sum2/2, Sum3/2
  Sum/1 -> Gain/1
  Sum3/1 -> Gain2/1
  Sum2/1 -> Gain1/1
  Sum1/1 -> Gain3/1

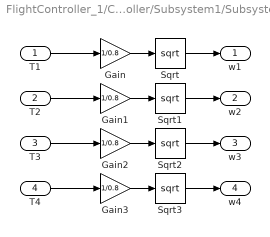
== system FlightController_1/Controller/Subsystem1/Subsystem1 ==
  T1 : Inport
  T2 : Inport  Port=2
  T3 : Inport  Port=3
  T4 : Inport  Port=4
  Gain{,1..3} (4 alike) : Gain  Gain=1/0.8
  Sqrt{,1..3} (4 alike) : Sqrt
  w1 : Outport
  w2 : Outport  Port=2
  w3 : Outport  Port=3
  w4 : Outport  Port=4
  wires:
  T1/1 -> Gain/1
  T2/1 -> Gain1/1
  T3/1 -> Gain2/1
  T4/1 -> Gain3/1
  Gain3/1 -> Sqrt3/1
  Gain2/1 -> Sqrt2/1
  Gain/1 -> Sqrt/1
  Gain1/1 -> Sqrt1/1
  Sqrt/1 -> w1/1
  Sqrt1/1 -> w2/1
  Sqrt2/1 -> w3/1
  Sqrt3/1 -> w4/1

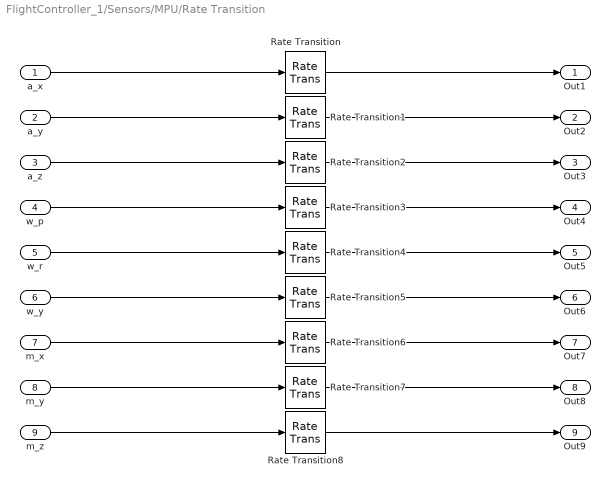
== system FlightController_1/Sensors/MPU/Rate Transition ==
  a_x : Inport
  a_y : Inport  Port=2
  a_z : Inport  Port=3
  w_p : Inport  Port=4
  w_r : Inport  Port=5
  w_y : Inport  Port=6
  m_x : Inport  Port=7
  m_y : Inport  Port=8
  m_z : Inport  Port=9
  Rate Transition{,1..8} (9 alike) : RateTransition  OutPortSampleTime=0.1
  Out1 : Outport
  Out2 : Outport  Port=2
  Out3 : Outport  Port=3
  Out4 : Outport  Port=4
  Out5 : Outport  Port=5
  Out6 : Outport  Port=6
  Out7 : Outport  Port=7
  Out8 : Outport  Port=8
  Out9 : Outport  Port=9
  wires:
  a_x/1 -> Rate Transition/1
  Rate Transition/1 -> Out1/1
  a_y/1 -> Rate Transition1/1
  Rate Transition1/1 -> Out2/1
  a_z/1 -> Rate Transition2/1
  Rate Transition2/1 -> Out3/1
  w_p/1 -> Rate Transition3/1
  Rate Transition3/1 -> Out4/1
  w_r/1 -> Rate Transition4/1
  Rate Transition4/1 -> Out5/1
  w_y/1 -> Rate Transition5/1
  Rate Transition5/1 -> Out6/1
  m_x/1 -> Rate Transition6/1
  Rate Transition6/1 -> Out7/1
  m_y/1 -> Rate Transition7/1
  Rate Transition7/1 -> Out8/1
  m_z/1 -> Rate Transition8/1
  Rate Transition8/1 -> Out9/1

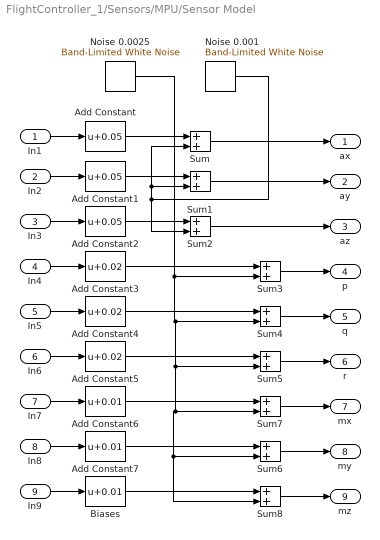
== system FlightController_1/Sensors/MPU/Sensor Model ==
  In1 : Inport
  In2 : Inport  Port=2
  In3 : Inport  Port=3
  In4 : Inport  Port=4
  In5 : Inport  Port=5
  In6 : Inport  Port=6
  In7 : Inport  Port=7
  In8 : Inport  Port=8
  In9 : Inport  Port=9
  Add Constant : Bias  Bias=0.05  SaturateOnIntegerOverflow=off
  Add Constant1 : Bias  Bias=0.05  SaturateOnIntegerOverflow=off
  Add Constant2 : Bias  Bias=0.05  SaturateOnIntegerOverflow=off
  Add Constant3 : Bias  Bias=0.02  SaturateOnIntegerOverflow=off
  Add Constant4 : Bias  Bias=0.02  SaturateOnIntegerOverflow=off
  Add Constant5 : Bias  Bias=0.02  SaturateOnIntegerOverflow=off
  Add Constant6 : Bias  Bias=0.01  SaturateOnIntegerOverflow=off
  Add Constant7 : Bias  Bias=0.01  SaturateOnIntegerOverflow=off
  Biases : Bias  Bias=0.01  SaturateOnIntegerOverflow=off
  Noise 0.001 : simulink/Sources/Band-Limited White Noise  Cov=[0.001]  Ts=0.1  seed=[23341]
  Noise 0.0025 : simulink/Sources/Band-Limited White Noise  Cov=[0.0025]  Ts=0.1  seed=[23341]
  Sum{,1..8} (9 alike) : Sum
  ax : Outport
  ay : Outport  Port=2
  az : Outport  Port=3
  p : Outport  Port=4
  q : Outport  Port=5
  r : Outport  Port=6
  mx : Outport  Port=7
  my : Outport  Port=8
  mz : Outport  Port=9
  wires:
  In1/1 -> Add Constant/1
  In2/1 -> Add Constant1/1
  In3/1 -> Add Constant2/1
  In4/1 -> Add Constant3/1
  In5/1 -> Add Constant4/1
  In6/1 -> Add Constant5/1
  In7/1 -> Add Constant6/1
  In8/1 -> Add Constant7/1
  In9/1 -> Biases/1
  Add Constant/1 -> Sum/1
  Noise 0.001/1 -> Sum/2, Sum1/2, Sum2/2
  Add Constant1/1 -> Sum1/1
  Add Constant2/1 -> Sum2/1
  Add Constant3/1 -> Sum3/1
  Noise 0.0025/1 -> Sum8/2, Sum6/2, Sum7/2, Sum5/2, Sum4/2, Sum3/2
  Add Constant4/1 -> Sum4/1
  Add Constant5/1 -> Sum5/1
  Add Constant7/1 -> Sum6/1
  Add Constant6/1 -> Sum7/1
  Biases/1 -> Sum8/1
  Sum/1 -> ax/1
  Sum2/1 -> az/1
  Sum1/1 -> ay/1
  Sum3/1 -> p/1
  Sum4/1 -> q/1
  Sum5/1 -> r/1
  Sum7/1 -> mx/1
  Sum6/1 -> my/1
  Sum8/1 -> mz/1

== matlab function FlightController_1/Sensors/MPU/Estimator ==
  data: ax input; phi output; ay input; az input; p input; q input; r input; mx input; my input; mz input; dt input; theta output; psi output
function [phi,theta,psi] = Estimator(ax,ay,az,p,q,r,mx,my,mz,dt)
% Complementary IMU filter (accel+gyro+mag). Inputs are measured
% accel (m/s^2), gyro (rad/s), mag (uT or any units), dt (s).
% Outputs: phi,theta,psi (rad)
% Tune: alpha (roll/pitch), beta (yaw trust)

% persistent states
persistent phi_hat theta_hat psi_hat
if isempty(phi_hat)
  phi_hat = 0; theta_hat = 0; psi_hat = 0;
end

% tuning (tweak)
alpha = 0.985;   % roll/pitch gyro trust (0.98-0.995 typical at 100-200Hz)
beta  = 0.98;    % yaw fusion gain for mag
g = 9.80665;
mag_expected = 45; % expected mag magnitude (uT) - tune to your world
tol_acc = 0.35*g;  % accel validity threshold
tol_mag = 0.4*mag_expected; % mag validity threshold (40%)

% 1) normalize / sanity checks
acc_norm = sqrt(ax*ax + ay*ay + az*az);
mag_norm = sqrt(mx*mx + my*my + mz*mz);

use_acc = (abs(acc_norm - g) < tol_acc) && (acc_norm>0.001);
use_mag = (abs(mag_norm - mag_expected) < tol_mag) && (mag_norm>0.001);

% 2) accel-based tilt (only if sane)
if use_acc
  phi_acc   = atan2( ay, az );
  theta_acc = atan2( -ax, sqrt(ay*ay + az*az) );
else
  phi_acc   = phi_hat;   % fallback: keep previous
  theta_acc = theta_hat;
end

% 3) gyro-based prediction
phi_pred   = phi_hat   + p*dt;
theta_pred = theta_hat + q*dt;
psi_pred   = psi_hat   + r*dt;

% 4) tilt-compensated mag heading (if mag ok)
if use_mag
  % use the current (predicted) roll/pitch for compensation (or use fused)
  cp = cos(theta_pred); sp = sin(theta_pred);
  cr = cos(phi_pred);   sr = sin(phi_pred);
  Xh = mx*cp + my*sr*sp + mz*cr*sp;
  Yh = my*cr - mz*sr;
  psi_mag = atan2(-Yh, Xh);  % adjust sign if your yaw convention differs
  % unwrap to avoid large jumps (make psi_mag near psi_pred)
  psi_mag = wrapToPi(psi_mag);
else
  psi_mag = psi_pred;
end

% 5) complementary fusion
phi_hat   = alpha*phi_pred   + (1-alpha)*phi_acc;
theta_hat = alpha*theta_pred + (1-alpha)*theta_acc;

% For yaw: if mag is valid fuse, otherwise pure gyro integration
if use_mag
  % handle wrap-around properly
  % ensure psi_pred and psi_mag are continuous
  d = wrapToPi(psi_mag - psi_pred);
  psi_hat = psi_pred + (1-beta)*d; % equivalent to beta*psi_pred + (1-beta)*psi_mag with wrap
else
  psi_hat = psi_pred;
end

% 6) return
phi = wrapToPi(phi_hat);
theta = wrapToPi(theta_hat);
psi = wrapToPi(psi_hat);

end

% helper: wrap to [-pi,pi]
function ang = wrapToPi(a)
 ang = mod(a+pi, 2*pi) - pi;
end

== matlab function FlightController_1/Plant/MATLAB Function1 ==
  settings: updateMethod=DISCRETE
  data: motor_rps input; acc_x output; acc_y output; acc_z output; gyro_x output; gyro_y output; gyro_z output; mag_x output; mag_y output; mag_z output; alt output
function [acc_x, acc_y, acc_z, gyro_x, gyro_y, gyro_z, mag_x, mag_y, mag_z, alt] = quadcopter_plant(motor_rps)
    %#codegen
    % Inputs:
    %   motor_rps: [4x1] motor speeds (rps)
    % Outputs:
    %   acc_x, acc_y, acc_z (accelerometer)
    %   gyro_x, gyro_y, gyro_z (gyroscope)
    %   mag_x, mag_y, mag_z (magnetometer)
    %   alt (altitude)

    % Physical constants
    m = 1.2;                % Mass (kg)
    g = 9.81;               % gravity (m/s^2)
    I = diag([0.014,0.018,0.028]); % inertia (kg*m^2)
    l = 0.225;              % arm length (m)
    b = 2.98e-6*(2*pi)^2;   % thrust coefficient
    d = 1.14e-7*(2*pi)^2;   % torque coefficient
    Cd = 0.1;               % drag coefficient
    m_e = [20; 0; -40];     % earth mag field (uT)
    wind = [0.5; 0; 0];     % wind vector (m/s)
    dt = 0.0001;

    % Persistent states
    persistent pos vel q omega
    if isempty(pos)
        pos   = [0;0;0];
        vel   = [0;0;0];
        q     = [1;0;0;0]; % quaternion [w;x;y;z]
        omega = [0;0;0];
    end

    q = q / norm(q); % Normalize quaternion

    % Motor to thrust
    omega_rot = 2*pi*motor_rps(:);       % rad/s
    T_i = b .* (omega_rot.^2);           % Thrust per motor

    % Torques
    tau_phi   = l * b * (T_i(2) - T_i(4));
    tau_theta = l * b * (T_i(3) - T_i(1));
    tau_psi   = d * (omega_rot(1)^2 - omega_rot(2)^2 + omega_rot(3)^2 - omega_rot(4)^2);
    tau = [tau_phi; tau_theta; tau_psi];

    % Net thrust in body frame
    F_thrust_b = [0; 0; sum(T_i)];

    % Rotate to inertial
    R = quat_to_rotmat(q);

    % Aerodynamic drag (in inertial frame)
    v_rel = vel - wind;
    F_drag_inertial = -Cd * v_rel;

    % Net acceleration in inertial frame
    g_vec = [0;0;-g];
    acc_inertial = (R * F_thrust_b + m * g_vec + F_drag_inertial) / m;

    % Quaternion kinematics
    Omega = [ 0    -omega(1) -omega(2) -omega(3);
              omega(1)  0     omega(3) -omega(2);
              omega(2) -omega(3)  0     omega(1);
              omega(3)  omega(2) -omega(1)  0 ];
    qdot = 0.5 * Omega * q;

    % Rotational dynamics
    omegadot = I \ (tau - cross(omega, I*omega));

    % Euler integration
    pos   = pos   + dt * vel;
    vel   = vel   + dt * acc_inertial;
    q     = q     + dt * qdot;
    omega = omega + dt * omegadot;
    q     = q / norm(q);

    % ---- Outputs ----
    a_b_true     = R' * (acc_inertial - g_vec); % Accelerometer in body frame
    omega_b_true = omega;                       % Gyroscope in body frame
    m_b_true     = R' * m_e;                    % Magnetometer in body frame
    alt          = pos(3);                      % Altitude (inertial z)

    % Split outputs to scalars
    acc_x = a_b_true(1);
    acc_y = a_b_true(2);
    acc_z = a_b_true(3);

    gyro_x = omega_b_true(1);
    gyro_y = omega_b_true(2);
    gyro_z = omega_b_true(3);

    mag_x = m_b_true(1);
    mag_y = m_b_true(2);
    mag_z = m_b_true(3);

    % Altitude is already scalar
end

function R = quat_to_rotmat(q)
    % Convert quaternion [w;x;y;z] to rotation matrix
    q0 = q(1); q1 = q(2); q2 = q(3); q3 = q(4);
    R = [ q0^2+q1^2-q2^2-q3^2,   2*(q1*q2 - q0*q3),     2*(q1*q3 + q0*q2);
          2*(q1*q2 + q0*q3),     q0^2-q1^2+q2^2-q3^2,   2*(q2*q3 - q0*q1);
          2*(q1*q3 - q0*q2),     2*(q2*q3 + q0*q1),     q0^2-q1^2-q2^2+q3^2 ];
end
